simulink model "sinus"  (R2013a)
settings: Solver=ode45  StartTime=0.0  StopTime=10.0  MaxStep=0.01  RelTol=1e-3
settings Model: Creator=Junior  LastModifiedBy=Dawid Perdek

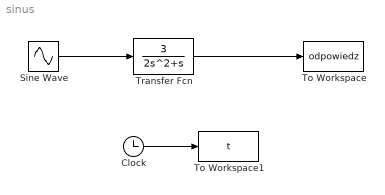
== system sinus ==
  Clock : Clock
  Sine Wave : Sin  Amplitude=4  Frequency=2  SampleTime=0
  To Workspace : ToWorkspace  VariableName=odpowiedz  SampleTime=-1
  To Workspace1 : ToWorkspace  VariableName=t  SampleTime=-1
  Transfer Fcn : TransferFcn  Numerator=[3]  Denominator=[2 1 0]
  wires:
  Sine Wave/1 -> Transfer Fcn/1
  Transfer Fcn/1 -> To Workspace/1
  Clock/1 -> To Workspace1/1
